simulink model "motor2"  (R2013a)
settings: Solver=ode45  StartTime=0.0  StopTime=10.0  RelTol=1e-3
values from neighbouring files (symbols this model uses):
  b = 0.1    [data_ideal_motor_1.mat]    (also in identificacion2.m)
  id_motor =     [LAB02_IDENT.mat]    (also in LAB02_IDENT_02.mat; data_ideal_motor_1.mat)
  J = 0.01    [data_ideal_motor_1.mat]    (also in identificacion2.m)
  K = K1    (= 1.59952738349)    [bodes.m]    (also in data_ideal_motor_1.mat = 0.01; identificacion2.m = 0.01)
  L = 0.5    [data_ideal_motor_1.mat]    (also in identificacion2.m)
  R = 1    [data_ideal_motor_1.mat]    (also in identificacion2.m)
libraries: dsparch4 x1
settings Model: Creator=u_labelectro  LastModifiedBy=u_labelectro

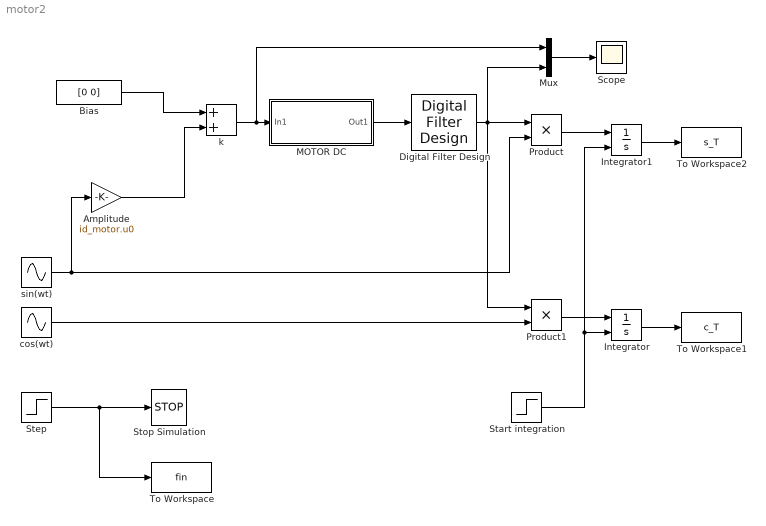
== system motor2 ==
  Amplitude : Gain  Gain=id_motor.u0
  Bias : FromWorkspace  VariableName=[0 0]  OutDataTypeStr=double  SampleTime=0
  Digital Filter Design : dsparch4/Digital Filter Design  mwdsp_browser_bugfix_var=off
  Integrator : Integrator  ExternalReset=rising
  Integrator1 : Integrator  ExternalReset=rising
  "MOTOR DC " : Subsystem  TreatAsAtomicUnit=on
  Mux : Mux  Inputs=2
  Product : Product
  Product1 : Product
  Scope : Scope
      settings: TimeRange=10
  Start integration : Step  Time=id_motor.Tstart  SampleTime=0
  Step : Step  Time=id_motor.Tstop  SampleTime=0
  Stop Simulation : Stop
  To Workspace : ToWorkspace  VariableName=fin  SampleTime=-1  SaveFormat=Timeseries
  To Workspace1 : ToWorkspace  VariableName=c_T  SampleTime=-1  SaveFormat=Timeseries
  To Workspace2 : ToWorkspace  VariableName=s_T  SampleTime=-1  SaveFormat=Timeseries
  cos(wt) : Sin  Phase=pi/2  Samples=id_motor.w  SampleTime=id_motor.s
  k : Sum
  sin(wt) : Sin  Frequency=id_motor.w  Samples=id_motor.w  SampleTime=id_motor.s
  wires:
  Step/1 -> To Workspace/1, Stop Simulation/1
  Bias/1 -> k/1
  Amplitude/1 -> k/2
  Digital Filter Design/1 -> Mux/2, Product/1, Product1/1
  "MOTOR DC "/1(Out1) -> Digital Filter Design/1
  k/1 -> Mux/1, "MOTOR DC "/1(In1)
  Product/1 -> Integrator1/1
  Product1/1 -> Integrator/1
  Start integration/1 -> Integrator/2, Integrator1/2
  sin(wt)/1 -> Amplitude/1, Product/2
  cos(wt)/1 -> Product1/2
  Integrator1/1 -> To Workspace2/1
  Integrator/1 -> To Workspace1/1
  Mux/1 -> Scope/1

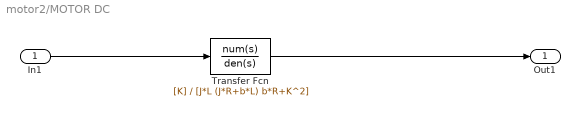
== system motor2/MOTOR DC  ==
  In1 : Inport
  Transfer Fcn : TransferFcn  Numerator=[K]  Denominator=[J*L (J*R+b*L) b*R+K^2]
  Out1 : Outport
  wires:
  Transfer Fcn/1 -> Out1/1
  In1/1 -> Transfer Fcn/1
